simulink model "REG1_submodel"  (R2020a)
settings: Solver=VariableStepAuto  StartTime=0.0  StopTime=10.0  RelTol=1e-3
model workspace (MAT data in the model file):
  D1_podbor1 = 902.0676
  D1_podbor_psi = 334.133298018
  D1_podbor_y = 97.9069
  D_podbor_x = 10
  D_podbor_z = 10
  I1_podbor1 = 320.9285
  I1_podbor_psi = 2.71828630961
  I1_podbor_y = 0.6752
  I_podbor_x = 50
  I_podbor_z = 50
  P1_podbor1 = 7509.4
  P1_podbor_psi = 848.547345881
  P1_podbor_y = 264.9363
  P_podbor_x = 50
  P_podbor_z = 50
  theta_1_P_param = Simulink.Parameter
  theta_1_P_param.Value = 1
  theta_1_P_param.DataType = 'auto'
  theta_1_P_param.Dimensions = [1 1]
  theta_1_P_paramCopy = Simulink.Parameter
  theta_1_P_paramCopy.Value = 1
  theta_1_P_paramCopy.DataType = 'auto'
  theta_1_P_paramCopy.Dimensions = [1 1]
undefined symbols (not defined in the file or in its folder): MAV, setup_pid
libraries: simulink x26, checkpacklib x2, dspsigattribs x1
settings Model: Creator=Tamer  LastModifiedBy=Tamer
settings SolverCC: ZeroCrossControl=DisableAll
settings DataIOCC: SaveOutput=off  SaveTime=off
settings GRTTargetCC: CombineOutputUpdateFcns=off  MatFileLogging=off

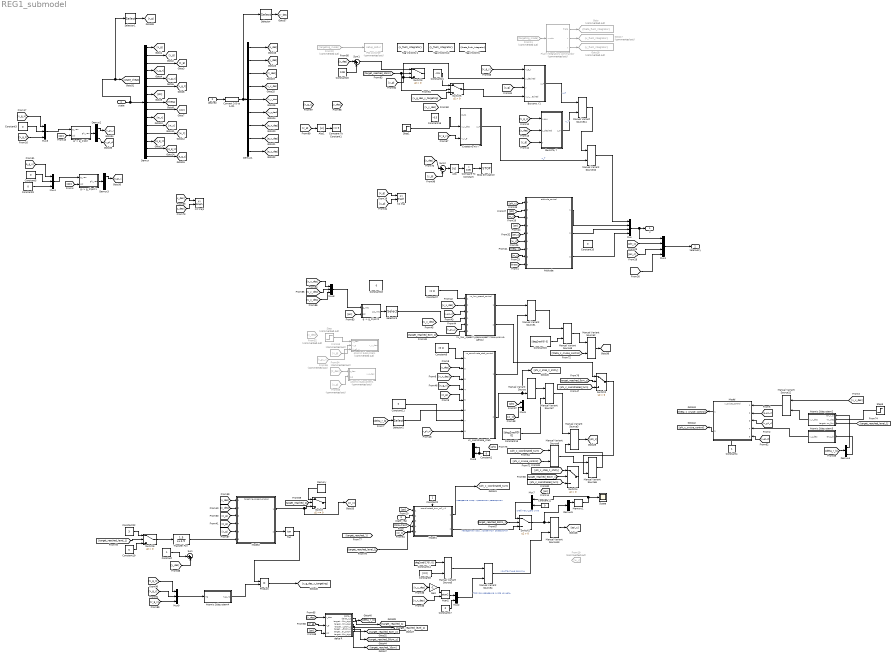
== system REG1_submodel ==
  state : Inport
  desired : Inport  Port=2  PortDimensions=[3, 3]
  state_real : Inport  Port=3
  Abs : Abs
  Abs1 : Abs
  Atan2 : Trigonometry  Operator=atan2
  Atomic Subsystem : Subsystem  Commented=on  TreatAsAtomicUnit=on
  Atomic Subsystem1 : Subsystem  Commented=on  TreatAsAtomicUnit=on
  Atomic Subsystem2 : Subsystem  TreatAsAtomicUnit=on
  Atomic Subsystem3 : Subsystem  TreatAsAtomicUnit=on
  Atomic Subsystem4 : Subsystem  TreatAsAtomicUnit=on
  Attitude : ModelReference  ModelNameDialog=attitude_control.slx  SimulationMode=Normal  ModelReferenceVersion=1.4
      settings: PortSchema="{\"entries\":[{\"content\":{\"sides\":[{\"content\":{\"connectorIds\":[\"In1\",\"In3\",\"In2\",\"In5\",\"In6\",\"In4\",\"In7\",\"In8\",\"In9\"]},\"type\":\"ConnectorPlacement.EquallySpacedRectSide\",\"uuid\":\"dbfcd847-4d65-4f0c-929f-179268b7fffa\"},{\"content\":{\"connectorIds\":[\"Out1\",\"Out2\",\"Out3\"],\"side\":\"RIGHT\"},\"type\":\"ConnectorPlacement.EquallySpacedRectSide\",\"uuid\":\"137158cb-e778-43b1-aea9-7a9702fa9882\"},{\"content\":{\"connectorIds\":[],\"side\":\"TOP\"},\"type\":\"ConnectorPlacement.EquallySpacedRectSide\",\"uuid\":\"f273673a-c2d4-42d6-9618-744ed2053ba7\"}]},\"type\":\"ConnectorPlacement.EquallySpacedConnector\",\"uuid\":\"b65e5f15-660d-4a08-8639-804897e62202\"}],\"packageUris\":[\"http://schema.mathworks.com/mf0/Connector/19700101\"],\"version\":\"1.0\"}"
  Compare To Constant : simulink/Logic and Bit Operations/Compare To Constant  relop=<  const=0.05  OutDataTypeStr=boolean
  Compare To Constant1 : simulink/Logic and Bit Operations/Compare To Constant  relop=<=  const=6  OutDataTypeStr=boolean
  Constant : Constant
  Constant{1,3,5,9..12,17..18} (9 alike) : Constant  Value=0
  Constant13 : Constant  Value=[deg2rad(0) 0]
  Constant14 : Constant  Value=[deg2rad(170); 0]
  Constant15 : Constant  Value=[deg2rad(0) 0]
  Constant16 : Constant  Value=-0.5
  Constant19 : Constant  Value=5
  Constant2 : Constant
  Constant20 : Constant  Value=0.08
  Constant21 : Constant  Value=-0.5
  Constant22 : Constant  Value=3
  Constant4 : Constant
  Constant6 : Constant  Value=[0 1]
  Constant7 : Constant  Value=[1 1]
  Constant8 : Constant  Value=[0 0]
  Convert 2-D to 1-D1 : dspsigattribs/Convert 2-D to 1-D
      settings: SourceProductBaseCode=DS
  Demux : Demux  Outputs=15
  Demux1 : Demux  Outputs=9
  Demux2 : Demux  Outputs=3
  Demux3 : Demux  Outputs=3
  Demux4 : Demux  Outputs=3
  Demux5 : Demux  Outputs=2
  Flush integrators commandor : Subsystem  Commented=on
  From11 : From  Commented=on  GotoTag=targeting_mode  TagVisibility=global
  From19 : From  Commented=on  GotoTag=w_y
  From22 : From  Commented=on  GotoTag=targeting_mode  TagVisibility=global
  From52 : From  Commented=on  GotoTag=x_des
  From53 : From  Commented=on  GotoTag=x_g
  From54 : From  Commented=on  GotoTag=z_des
  From55 : From  Commented=on  GotoTag=z_g
  From56 : From  Commented=on  GotoTag=v_g1_x
  Gain : Gain  Gain=-1
  Goto : Goto  Commented=on  GotoTag=theta_flush_integrator  TagVisibility=scoped
  Goto17 : Goto  Commented=on  GotoTag=x_flush_integrator  TagVisibility=scoped
  Goto18 : Goto  Commented=on  GotoTag=y_flush_integrator  TagVisibility=scoped
  Manual Variant Source{,1,4,7..8,10..11,13} (8 alike) : simulink/Signal Routing/Manual Variant Source  NumChoices=2  LabelModeActiveChoice=V_1
  Manual Variant Source{2..3,5..6,9,12} (6 alike) : simulink/Signal Routing/Manual Variant Source  NumChoices=2  LabelModeActiveChoice=V_2
  Memory : Memory
  Memory1 : Memory
  Model : ModelReference  ModelNameDialog=v_cruise_control.slx  SimulationMode=Normal  ModelReferenceVersion=1.37  EnablePortName=Enable  EnablePortStatesWhenEnabling=held
  Model1 : ModelReference  ModelNameDialog=coordinated_turn_roll_v1.slx  SimulationMode=Normal  ModelReferenceVersion=1.128  EnablePortName=Enable  EnablePortStatesWhenEnabling=held
  Model2 : ModelReference  ModelNameDialog=targeting_speed_angles.slx  SimulationMode=Normal  ModelReferenceVersion=1.18
  Mux : Mux
  Mux1 : Mux
  Mux{2,5..7} (4 alike) : Mux  Inputs=2
  Mux{3..4,8..9} (4 alike) : Mux  Inputs=3
  PID switcher : MATLABFcn  Commented=on  MATLABFcn=setup_pid(u)  OutputDimensions=0  Output1D=off
  Product : Product
  Scope : Scope
  Selector : Selector  InputPortWidth=9  IndexOptions=Index vector (dialog)  Indices=[1:3]  OutputSizes=1
  Selector1 : Selector  InputPortWidth=15  IndexOptions=Index vector (dialog)  Indices=[1:3]  OutputSizes=1
  Selector2 : Selector  InputPortWidth=3  IndexOptions=Index vector (dialog)  Indices=[3]  OutputSizes=1
  Selector3 : Selector  InputPortWidth=3  IndexOptions=Index vector (dialog)  Indices=[3]  OutputSizes=1
  Step : Step  Commented=on  Time=0.2  After=5  SampleTime=0
  Step1 : Step  Time=3  Before=-1  After=0  SampleTime=0
  Step3 : Step  Time=0  After=20  SampleTime=0
  Stop Simulation : Stop
  Sum : Sum  Inputs=|++
  Sum1 : Sum  Inputs=|++
  Sum2 : Sum  Inputs=|+-
  Switch : Switch  Criteria=u2 ~= 0
  Switch{1..6} (6 alike) : Switch  Criteria=u2 > Threshold
  Tag Visibility : GotoTagVisibility  GotoTag=theta_flush_integrator
  Tag Visibility1 : GotoTagVisibility  GotoTag=x_flush_integrator
  Tag Visibility2 : GotoTagVisibility  GotoTag=y_flush_integrator
  Tan : Trigonometry  Operator=tan
  Transfer Fcn : TransferFcn  Numerator=[1.5]  Denominator=[1 1.5]
  XZ traj : simulink/Sinks/XY Graph  xmin=-2  xmax=20  ymin=-2  ymax=20  st=-1
  XZ traj1 : simulink/Sinks/XY Graph  xmin=20  xmax=80  ymin=20  ymax=80  st=-1
  delta R : Subsystem  TreatAsAtomicUnit=on
  "g -> g_1(psi)" : MATLAB Function  TreatAsAtomicUnit=on
  "g -> g_1(psi)1" : MATLAB Function  TreatAsAtomicUnit=on
  "g -> g_1(psi)2" : MATLAB Function  TreatAsAtomicUnit=on
  xz_coordinate_stab : ModelReference  ModelNameDialog=xz_coordinate_stab_control.slx  SimulationMode=Normal  ModelReferenceVersion=1.10
  zx_low_speed (удерживает позицию на ветру) : ModelReference  ModelNameDialog=xz_low_speed_control.slx  SimulationMode=Normal  ModelReferenceVersion=1.12
  "Высота, Y" : Subsystem
      settings: PortSchema="{\"entries\":[{\"content\":{\"sides\":[{\"content\":{\"connectorIds\":[]},\"type\":\"ConnectorPlacement.EquallySpacedRectSide\",\"uuid\":\"a258f665-a86a-4482-bd07-3187ea478656\"},{\"content\":{\"connectorIds\":[],\"side\":\"RIGHT\"},\"type\":\"ConnectorPlacement.EquallySpacedRectSide\",\"uuid\":\"4cc1ffc1-e5d7-4190-ba75-89ce977e4acc\"},{\"content\":{\"connectorIds\":[\"Out1\"],\"side\":\"TOP\"},\"type\":\"ConnectorPlacement.EquallySpacedRectSide\",\"uuid\":\"daf9489c-9fb9-498c-b344-dda7a980194c\"},{\"content\":{\"connectorIds\":[\"In1\",\"In2\",\"In3\"],\"side\":\"BOTTOM\"},\"type\":\"ConnectorPlacement.EquallySpacedRectSide\",\"uuid\":\"f778d476-c858-4cc3-a786-5ff47391ec3b\"}]},\"type\":\"ConnectorPlacement.EquallySpacedConnector\",\"uuid\":\"5a79eedc-deb4-47bd-85cd-0d2cb0ea5802\"}],\"packageUris\":[\"http://schema.mathworks.com/mf0/Connector/19700101\"],\"version\":\"1.0\"}"
  "Высота, Y1" : Subsystem
      settings: PortSchema="{\"entries\":[{\"content\":{\"sides\":[{\"content\":{\"connectorIds\":[]},\"type\":\"ConnectorPlacement.EquallySpacedRectSide\",\"uuid\":\"a258f665-a86a-4482-bd07-3187ea478656\"},{\"content\":{\"connectorIds\":[],\"side\":\"RIGHT\"},\"type\":\"ConnectorPlacement.EquallySpacedRectSide\",\"uuid\":\"4cc1ffc1-e5d7-4190-ba75-89ce977e4acc\"},{\"content\":{\"connectorIds\":[\"Out1\"],\"side\":\"TOP\"},\"type\":\"ConnectorPlacement.EquallySpacedRectSide\",\"uuid\":\"daf9489c-9fb9-498c-b344-dda7a980194c\"},{\"content\":{\"connectorIds\":[\"In1\",\"In2\",\"In3\",\"In4\"],\"side\":\"BOTTOM\"},\"type\":\"ConnectorPlacement.EquallySpacedRectSide\",\"uuid\":\"f778d476-c858-4cc3-a786-5ff47391ec3b\"}]},\"type\":\"ConnectorPlacement.EquallySpacedConnector\",\"uuid\":\"5a79eedc-deb4-47bd-85cd-0d2cb0ea5802\"}],\"packageUris\":[\"http://schema.mathworks.com/mf0/Connector/19700101\"],\"version\":\"1.0\"}"
  Скорость по Y : Subsystem
      settings: PortSchema="{\"entries\":[{\"content\":{\"sides\":[{\"content\":{\"connectorIds\":[]},\"type\":\"ConnectorPlacement.EquallySpacedRectSide\",\"uuid\":\"a258f665-a86a-4482-bd07-3187ea478656\"},{\"content\":{\"connectorIds\":[],\"side\":\"RIGHT\"},\"type\":\"ConnectorPlacement.EquallySpacedRectSide\",\"uuid\":\"4cc1ffc1-e5d7-4190-ba75-89ce977e4acc\"},{\"content\":{\"connectorIds\":[\"Out2\"],\"side\":\"TOP\"},\"type\":\"ConnectorPlacement.EquallySpacedRectSide\",\"uuid\":\"daf9489c-9fb9-498c-b344-dda7a980194c\"},{\"content\":{\"connectorIds\":[\"Out1\",\"In1\",\"In2\"],\"side\":\"BOTTOM\"},\"type\":\"ConnectorPlacement.EquallySpacedRectSide\",\"uuid\":\"f778d476-c858-4cc3-a786-5ff47391ec3b\"}]},\"type\":\"ConnectorPlacement.EquallySpacedConnector\",\"uuid\":\"5a79eedc-deb4-47bd-85cd-0d2cb0ea5802\"}],\"packageUris\":[\"http://schema.mathworks.com/mf0/Connector/19700101\"],\"version\":\"1.0\"}"
  u : Outport
  telemetry : Outport  Port=2
  wires:
  desired/1 -> Convert 2-D to 1-D1/1
  Demux/4 -> [v_g_x]
  Demux/15 -> [a_g_z]
  Demux/13 -> [a_g_x]
  Demux/12 -> [w_z]
  From22/1 -> PID switcher/1
  Demux/3 -> [z_g]
  Demux/6 -> [v_g_z]
  Demux1/1 -> [x_des]
  Demux1/4 -> [v_x_des]
  Demux/5 -> [v_g_y]
  Demux/2 -> [y_g]
  Demux/1 -> [x_g]
  Mux/1 -> Mux1/1, u/1
  Flush integrators commandor/1(theta) -> Goto/1
  Convert 2-D to 1-D1/1 -> Selector/1, Demux1/1
  Flush integrators commandor/3(y) -> Goto18/1
  Demux1/2 -> [y_des]
  Demux/14 -> [a_g_y]
  [psi_c] -> Mux1/3
  Demux/7 -> [phi]
  Demux1/5 -> [v_y_des]
  Constant3/1 -> Mux3/2
  Mux1/1 -> telemetry/1
  Demux1/8 -> [a_y_des]
  [psi] -> "g -> g_1(psi)"/2(psi)
  [phi_c] -> Mux1/2
  Demux1/6 -> [v_z_des]
  Mux3/1 -> "g -> g_1(psi)"/1(g_vec)
  Demux1/3 -> [z_des]
  Demux2/1 -> [v_g1_x]
  [v_g_z] -> Mux3/3
  Demux/10 -> [w_x]
  [v_g_x] -> Mux3/1
  Flush integrators commandor/2(x) -> Goto17/1
  "Высота, Y"/1(u_T) -> Manual Variant Source11/2  "u_T"
  Demux/8 -> [theta]
  Demux2/3 -> [v_g1_z]
  From11/1 -> Flush integrators commandor/1(mode)
  [y_g] -> "Высота, Y"/3(y)
  "g -> g_1(psi)"/1(g1_vec) -> Demux2/1
  Demux1/7 -> [a_x_des]
  Demux/9 -> [psi]
  [theta_c] -> Mux1/4
  Demux1/9 -> [a_z_des]
  Demux/11 -> [w_y]
  Constant7/1 -> zx_low_speed (удерживает позицию на ветру)/1
  [v_g_y] -> "Высота, Y"/1(v_g_y)
  [y_des] -> "Высота, Y"/2(y_desired)
  [v_g1_z] -> zx_low_speed (удерживает позицию на ветру)/5
  [v_g1_x] -> zx_low_speed (удерживает позицию на ветру)/3
  [v_x_des] -> xz_coordinate_stab/3
  [x_des] -> xz_coordinate_stab/2
  [x_g] -> xz_coordinate_stab/5
  [v_g_x] -> xz_coordinate_stab/4
  [v_g1_z] -> xz_coordinate_stab/8
  Constant6/1 -> xz_coordinate_stab/1
  xz_coordinate_stab/2 -> [phi_c_stab_z_shitly], Manual Variant Source/2
  xz_coordinate_stab/1 -> Manual Variant Source1/2
  zx_low_speed (удерживает позицию на ветру)/1 -> Manual Variant Source1/1
  [theta] -> Attitude/9
  [phi] -> Attitude/3
  [w_x] -> Attitude/2
  [phi_c] -> Attitude/1
  Attitude/1 -> Mux/2
  Attitude/3 -> Mux/4
  Constant4/1 -> Model/Enable
  Manual Variant Source2/1 -> [theta_c]
  [v_g1_x] -> Model/3
  Demux3/1 -> [a_g1_x]
  Constant9/1 -> Mux4/3
  [a_g_x] -> Mux4/1
  [psi] -> "g -> g_1(psi)1"/2(psi)
  Mux4/1 -> "g -> g_1(psi)1"/1(g_vec)
  Constant5/1 -> Mux4/2
  "g -> g_1(psi)1"/1(g1_vec) -> Demux3/1
  [a_g1_x] -> Model/2
  Attitude/2 -> Mux/3
  [psi] -> Model1/1
  state_real/1 -> Model1/2
  Constant2/1 -> Model1/Enable
  [psi] -> Attitude/5
  [psi_c] -> Attitude/6
  [w_y] -> Attitude/4
  [theta_c] -> Attitude/7
  [w_z] -> Attitude/8
  [x_g] -> XZ traj/1
  [z_g] -> XZ traj/2
  [v_z_des] -> Gain/1
  Gain/1 -> Atan2/1
  [v_x_des] -> Atan2/2
  Atan2/1 -> Mux2/1
  Mux2/1 -> Manual Variant Source4/2  "Прямое наведение курса на цель"
  state/1 -> Selector1/1, [state_cheat], Demux/1
  [w_x] -> Mux6/2
  [phi] -> Mux6/1
  Manual Variant Source/1 -> Manual Variant Source7/1
  Manual Variant Source7/1 -> Manual Variant Source3/1
  Constant13/1 -> Manual Variant Source7/2
  [state_cheat] -> Model1/3
  [x_des] -> Model2/1
  [z_des] -> Model2/2
  [z_g] -> Model2/4
  [x_g] -> Model2/3
  [xi_c] -> Model1/4
  From53/1 -> Atomic Subsystem/2(x_g)
  From55/1 -> Atomic Subsystem1/2(z_g)
  From54/1 -> Atomic Subsystem1/1(z_des)
  From56/1 -> Atomic Subsystem/3(V_g1_x)
  Atomic Subsystem3/1(v_z_des) -> Model/4
  [v_g1_z] -> Model/5
  Step/1 -> Atomic Subsystem/1(x_des)
  [v_x_des] -> zx_low_speed (удерживает позицию на ветру)/2
  [v_x_des] -> Manual Variant Source12/1
  Selector/1 -> [r_des]
  Selector1/1 -> [r_g]
  Model2/1 -> [xi_c], Switch/3
  Memory/1 -> Switch/1
  Model1/2 -> Switch1/3  "наведение координированным разворотом"
  Constant12/1 -> Mux7/2
  [target_reached_50cm_z] -> Switch1/2
  [delta_r_b] -> Demux4/1
  Demux4/3 -> Atomic Subsystem3/1(err_z_b)
  Demux4/1 -> Atomic Subsystem2/1(err_x_b)
  Manual Variant Source9/1 -> Manual Variant Source2/1
  Manual Variant Source1/1 -> Manual Variant Source9/1
  Constant15/1 -> Manual Variant Source9/2
  [v_g_y] -> Скорость по Y/2(v_y_g)
  Скорость по Y/2(u_T) -> Manual Variant Source10/2  "u_T"
  Manual Variant Source10/1 -> Mux/1
  Step1/1 -> Скорость по Y/1(v_y_des)
  [v_g_y] -> "Высота, Y1"/1(v_g_y)
  [y_g] -> "Высота, Y1"/3(y)
  "Высота, Y1"/1(u_T) -> Manual Variant Source11/1  "u_T"
  Manual Variant Source11/1 -> Manual Variant Source10/1
  Manual Variant Source12/1 -> Model/1
  Atomic Subsystem2/1(v_x_des) -> Manual Variant Source12/2
  Constant17/1 -> Mux2/2
  Constant14/1 -> Manual Variant Source5/1
  Constant8/1 -> Manual Variant Source5/2
  Manual Variant Source13/1 -> [psi_c]
  Manual Variant Source5/1 -> Manual Variant Source4/1
  Manual Variant Source4/1 -> Manual Variant Source13/2  "константные режимы"
  delta R/2(delta_r_b) -> [delta_r_b]
  [psi] -> delta R/3(psi)
  [r_des] -> delta R/1(r_des)
  [r_g] -> delta R/2(r_g)
  delta R/3(target_near_1.5m_sign) -> [target_reached_1]
  [target_reached_1] -> Switch/2
  [phi_c_coordinated_turn] -> Manual Variant Source8/1
  Model/2 -> [phi_c_cruise_control]
  [phi_c_cruise_control] -> Manual Variant Source8/2
  Manual Variant Source3/1 -> [phi_c]
  Model/1 -> [theta_c_cruise_control]
  [theta_c_cruise_control] -> Manual Variant Source2/2
  [x_des] -> XZ traj1/1
  [z_des] -> XZ traj1/2
  Step3/1 -> Atomic Subsystem2/2(Vx_des)
  delta R/4(target_near_3m_sign) -> [target_reached_level_1]
  [target_reached_level_1] -> Atomic Subsystem2/3(target_near_3m)
  Model1/1 -> [phi_c_coordinated_turn]  "наведение координированным разворотом"
  Constant1/1 -> Mux5/1, Mux5/2
  [target_reached_5cm_z] -> Switch2/2
  delta R/5(target_near_5cm_z) -> [target_reached_5cm_z]
  Mux7/1 -> Switch1/1  "стаб текущего угла"
  [target_reached_level_1] -> Model1/5
  Switch1/1 -> Demux5/1, Manual Variant Source13/1
  delta R/6(target_near_50cm_z) -> [target_reached_50cm_z]
  Manual Variant Source6/1 -> Manual Variant Source3/2
  Manual Variant Source8/1 -> Manual Variant Source6/1
  [target_reached_50cm_z] -> Switch4/2
  [phi_c_stab_z_shitly] -> Switch4/1
  [phi_c_coordinated_turn] -> Switch4/3
  Demux5/1 -> Memory1/1
  Memory1/1 -> Scope/1, Mux7/1
  Constant11/1 -> xz_coordinate_stab/7
  [delta_r_b] -> Selector2/1
  Selector2/1 -> xz_coordinate_stab/6
  zx_low_speed (удерживает позицию на ветру)/2 -> Switch2/1
  [phi_c_coordinated_turn] -> Switch2/3
  [target_reached_5cm_z] -> zx_low_speed (удерживает позицию на ветру)/6
  Switch2/1 -> Manual Variant Source6/2
  [psi] -> "g -> g_1(psi)2"/2(psi)
  [v_x_des] -> Mux8/1
  [v_y_des] -> Mux8/2
  [v_z_des] -> Mux8/3
  Mux8/1 -> "g -> g_1(psi)2"/1(g_vec)
  "g -> g_1(psi)2"/1(g1_vec) -> Selector3/1
  Selector3/1 -> zx_low_speed (удерживает позицию на ветру)/4
  [y_g] -> Model2/5
  [v_g_y] -> Mux9/2
  Mux9/1 -> Atomic Subsystem4/1(Vg)
  [v_g_z] -> Mux9/3
  [v_g_x] -> Mux9/1
  Model2/2 -> Tan/1
  Atomic Subsystem4/1(V_g_xz) -> Product/2
  Tan/1 -> Product/1
  Switch5/1 -> "Высота, Y1"/4(v_y_desired)
  [y_g] -> "Высота, Y1"/2(y_desired), Switch3/3
  [target_reached_10cm] -> Switch5/2, Switch3/2
  Sum1/1 -> Switch3/1
  [v_g_des_y_targeting] -> Switch5/3
  delta R/7(target_near_10cm) -> [target_reached_10cm]
  [y_des] -> Sum1/1
  Constant20/1 -> Sum1/2
  [y_des] -> Sum/2
  Constant/1 -> Sum/1
  Sum2/1 -> Abs/1
  [y_des] -> Sum2/1
  [y_g] -> Sum2/2
  Abs/1 -> Compare To Constant/1
  Constant21/1 -> Switch5/1
  Abs1/1 -> Compare To Constant1/1
  [y_g] -> Abs1/1
  Constant22/1 -> Switch6/1
  Constant19/1 -> Switch6/3
  [target_reached_level_1] -> Switch6/2
  Compare To Constant/1 -> Stop Simulation/1
  Switch6/1 -> Transfer Fcn/1
  Transfer Fcn/1 -> Model2/6
  Product/1 -> [v_g_des_y_targeting]

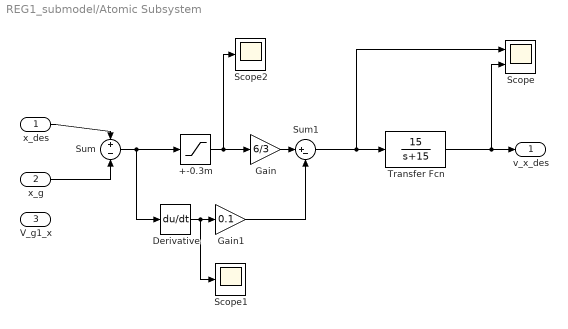
== system REG1_submodel/Atomic Subsystem ==
  x_des : Inport
  x_g : Inport  Port=2
  V_g1_x : Inport  Port=3
  +-0.3m : Saturate  UpperLimit=3  LowerLimit=-3
  Derivative : Derivative
  Gain : Gain  Gain=6/3
  Gain1 : Gain  Gain=0.1
  Scope : Scope  NumInputPorts=2
  Scope1 : Scope
  Scope2 : Scope
  Sum : Sum  Inputs=+-
  Sum1 : Sum  Inputs=|+-
  Transfer Fcn : TransferFcn  Numerator=[15]  Denominator=[1 15]
  v_x_des : Outport
  wires:
  x_des/1 -> Sum/1
  x_g/1 -> Sum/2
  +-0.3m/1 -> Scope2/1, Gain/1
  Gain/1 -> Sum1/1
  Sum1/1 -> Transfer Fcn/1, Scope/1
  Gain1/1 -> Sum1/2
  Sum/1 -> Derivative/1, +-0.3m/1
  Derivative/1 -> Scope1/1, Gain1/1
  Transfer Fcn/1 -> Scope/2, v_x_des/1

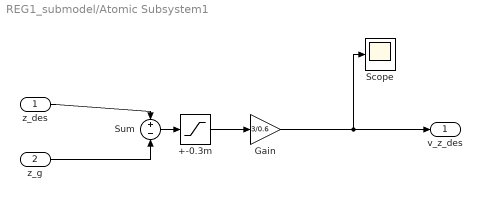
== system REG1_submodel/Atomic Subsystem1 ==
  z_des : Inport
  z_g : Inport  Port=2
  +-0.3m : Saturate  UpperLimit=0.6  LowerLimit=-0.6
  Gain : Gain  Gain=3/0.6
  Scope : Scope
  Sum : Sum  Inputs=+-
  v_z_des : Outport
  wires:
  z_des/1 -> Sum/1
  z_g/1 -> Sum/2
  Sum/1 -> +-0.3m/1
  +-0.3m/1 -> Gain/1
  Gain/1 -> Scope/1, v_z_des/1

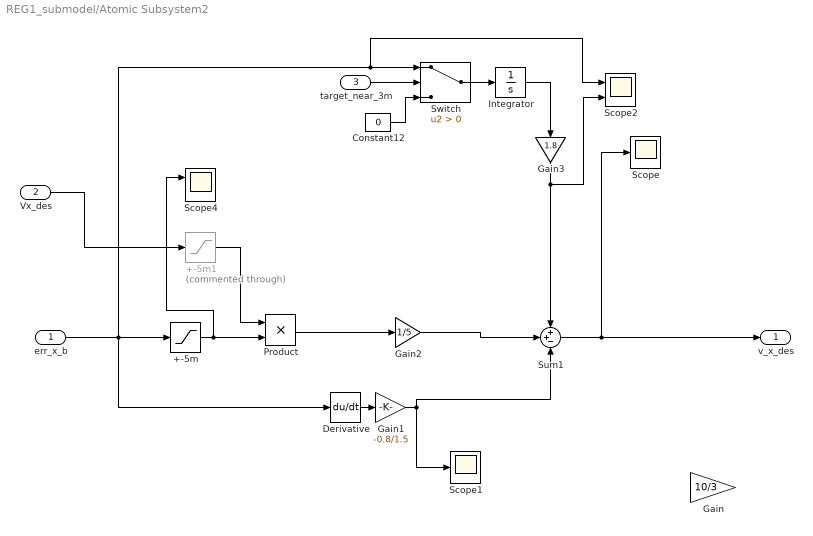
== system REG1_submodel/Atomic Subsystem2 ==
  err_x_b : Inport
  Vx_des : Inport  Port=2
  target_near_3m : Inport  Port=3
  +-5m : Saturate  UpperLimit=5  LowerLimit=-5
  +-5m1 : Saturate  Commented=through  UpperLimit=20  LowerLimit=-20
  Constant12 : Constant  Value=0
  Derivative : Derivative
  Gain : Gain  Gain=10/3
  Gain1 : Gain  Gain=-0.8/1.5
  Gain2 : Gain  Gain=1/5
  Gain3 : Gain  Gain=1.8
  Integrator : Integrator
  Product : Product
  Scope : Scope
  Scope1 : Scope
  Scope2 : Scope  NumInputPorts=2
  Scope4 : Scope  NumInputPorts=2
  Sum1 : Sum  Inputs=++-
  Switch : Switch  Criteria=u2 > Threshold
  v_x_des : Outport
  wires:
  +-5m/1 -> Scope4/1, Product/2
  err_x_b/1 -> Scope2/1, Switch/1, +-5m/1, Derivative/1
  Gain1/1 -> Sum1/3, Scope1/1
  Derivative/1 -> Gain1/1
  Product/1 -> Gain2/1
  Sum1/1 -> v_x_des/1, Scope/1
  target_near_3m/1 -> Switch/2
  Switch/1 -> Integrator/1
  Constant12/1 -> Switch/3
  Gain3/1 -> Sum1/1, Scope2/2
  Integrator/1 -> Gain3/1
  Gain2/1 -> Sum1/2
  Vx_des/1 -> +-5m1/1
  +-5m1/1 -> Product/1

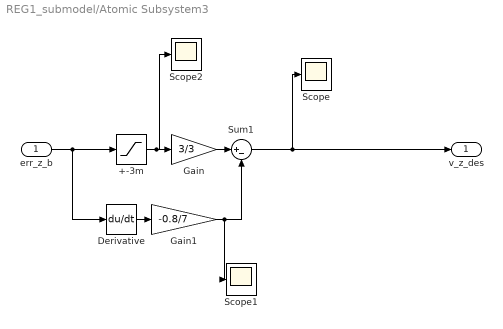
== system REG1_submodel/Atomic Subsystem3 ==
  err_z_b : Inport
  +-3m : Saturate  UpperLimit=3  LowerLimit=-3
  Derivative : Derivative
  Gain : Gain  Gain=3/3
  Gain1 : Gain  Gain=-0.8/7
  Scope : Scope
  Scope1 : Scope
  Scope2 : Scope
  Sum1 : Sum  Inputs=|+-
  v_z_des : Outport
  wires:
  +-3m/1 -> Scope2/1, Gain/1
  Gain/1 -> Sum1/1
  Sum1/1 -> v_z_des/1, Scope/1
  err_z_b/1 -> Derivative/1, +-3m/1
  Gain1/1 -> Sum1/2, Scope1/1
  Derivative/1 -> Gain1/1

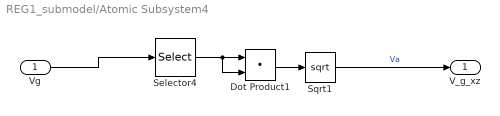
== system REG1_submodel/Atomic Subsystem4 ==
  Vg : Inport
  Dot Product1 : DotProduct  InputSameDT=on  OutDataTypeStr=Inherit: Inherit via internal rule
  Selector4 : Selector  InputPortWidth=3  IndexOptions=Index vector (dialog)  Indices=[1 3]  OutputSizes=1
  Sqrt1 : Sqrt  SaturateOnIntegerOverflow=on
  V_g_xz : Outport
  wires:
  Selector4/1 -> Dot Product1/2, Dot Product1/1
  Dot Product1/1 -> Sqrt1/1
  Vg/1 -> Selector4/1
  Sqrt1/1 -> V_g_xz/1  "Va"

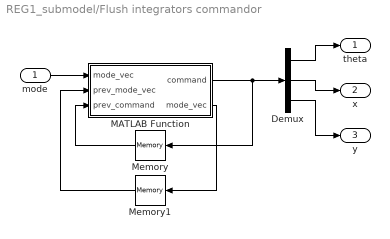
== system REG1_submodel/Flush integrators commandor ==
  mode : Inport
  Demux : Demux  Outputs=3
  MATLAB Function : MATLAB Function  TreatAsAtomicUnit=on
  Memory : Memory  InitialCondition=[0 0 0]'
  Memory1 : Memory  InitialCondition=[0 0]'
  theta : Outport
  x : Outport  Port=2
  y : Outport  Port=3
  wires:
  mode/1 -> MATLAB Function/1("mode_vec ")
  MATLAB Function/1(command) -> Memory/1, Demux/1
  Memory/1 -> MATLAB Function/3(prev_command)
  Demux/1 -> theta/1
  Demux/2 -> x/1
  Demux/3 -> y/1
  MATLAB Function/2(mode_vec) -> Memory1/1
  Memory1/1 -> MATLAB Function/2(prev_mode_vec)

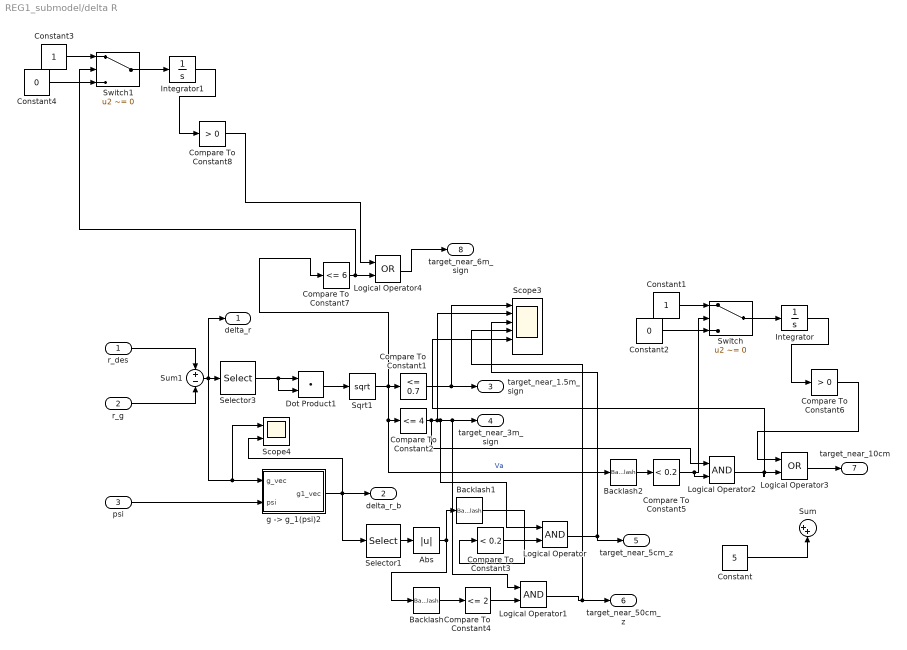
== system REG1_submodel/delta R ==
  r_des : Inport
  r_g : Inport  Port=2
  psi : Inport  Port=3
  Abs : Abs
  Backlash : Backlash  InitialOutput=2
  Backlash1 : Backlash  BacklashWidth=0.1  InitialOutput=0.2
  Backlash2 : Backlash  BacklashWidth=0.1  InitialOutput=0.25
  Compare To Constant1 : simulink/Logic and Bit Operations/Compare To Constant  relop=<=  const=0.7  OutDataTypeStr=boolean
  Compare To Constant2 : simulink/Logic and Bit Operations/Compare To Constant  relop=<=  const=4  OutDataTypeStr=boolean
  Compare To Constant3 : simulink/Logic and Bit Operations/Compare To Constant  relop=<  const=0.2  OutDataTypeStr=boolean
  Compare To Constant4 : simulink/Logic and Bit Operations/Compare To Constant  relop=<=  const=2  OutDataTypeStr=boolean
  Compare To Constant5 : simulink/Logic and Bit Operations/Compare To Constant  relop=<  const=0.2  OutDataTypeStr=boolean
  Compare To Constant6 : simulink/Logic and Bit Operations/Compare To Constant  relop=>  const=0  OutDataTypeStr=boolean
  Compare To Constant7 : simulink/Logic and Bit Operations/Compare To Constant  relop=<=  const=6  OutDataTypeStr=boolean
  Compare To Constant8 : simulink/Logic and Bit Operations/Compare To Constant  relop=>  const=0  OutDataTypeStr=boolean
  Constant : Constant  Value=5
  Constant1 : Constant
  Constant2 : Constant  Value=0
  Constant3 : Constant
  Constant4 : Constant  Value=0
  Dot Product1 : DotProduct  InputSameDT=on  OutDataTypeStr=Inherit: Inherit via internal rule
  Integrator : Integrator
  Integrator1 : Integrator
  Logical Operator : Logic  AllPortsSameDT=off  OutDataTypeStr=boolean
  Logical Operator1 : Logic  AllPortsSameDT=off  OutDataTypeStr=boolean
  Logical Operator2 : Logic  AllPortsSameDT=off  OutDataTypeStr=boolean
  Logical Operator3 : Logic  Operator=OR  AllPortsSameDT=off  OutDataTypeStr=boolean
  Logical Operator4 : Logic  Operator=OR  AllPortsSameDT=off  OutDataTypeStr=boolean
  Scope3 : Scope  NumInputPorts=6
  Scope4 : Scope  NumInputPorts=2
  Selector1 : Selector  InputPortWidth=3  IndexOptions=Index vector (dialog)  Indices=[3]  OutputSizes=1
  Selector3 : Selector  InputPortWidth=3  IndexOptions=Index vector (dialog)  Indices=[1 3]  OutputSizes=1
  Sqrt1 : Sqrt  SaturateOnIntegerOverflow=on
  Sum : Sum  Inputs=|++
  Sum1 : Sum  Inputs=+-
  Switch : Switch  Criteria=u2 ~= 0
  Switch1 : Switch  Criteria=u2 ~= 0
  "g -> g_1(psi)2" : MATLAB Function  TreatAsAtomicUnit=on
  delta_r : Outport
  delta_r_b : Outport  Port=2
  target_near_1.5m_sign : Outport  Port=3
  target_near_3m_sign : Outport  Port=4
  target_near_5cm_z : Outport  Port=5
  target_near_50cm_z : Outport  Port=6
  target_near_10cm : Outport  Port=7
  target_near_6m_sign : Outport  Port=8
  wires:
  r_g/1 -> Sum1/2
  Selector3/1 -> Dot Product1/2, Dot Product1/1
  Dot Product1/1 -> Sqrt1/1
  psi/1 -> "g -> g_1(psi)2"/2(psi)
  Sum1/1 -> delta_r/1, Selector3/1, Scope4/1, "g -> g_1(psi)2"/1(g_vec)
  Sqrt1/1 -> Compare To Constant7/1, Backlash2/1, Compare To Constant2/1, Compare To Constant1/1  "Va"
  "g -> g_1(psi)2"/1(g1_vec) -> Selector1/1, delta_r_b/1, Scope4/2
  r_des/1 -> Sum1/1
  Compare To Constant1/1 -> Scope3/1, target_near_1.5m_sign/1
  Compare To Constant2/1 -> Logical Operator2/1, target_near_3m_sign/1, Logical Operator1/1, Logical Operator/1, Scope3/2
  Selector1/1 -> Abs/1
  Logical Operator/1 -> target_near_5cm_z/1, Scope3/3
  Compare To Constant3/1 -> Logical Operator/2
  Compare To Constant4/1 -> Logical Operator1/2
  Logical Operator1/1 -> Scope3/4, target_near_50cm_z/1
  Abs/1 -> Backlash1/1, Backlash/1
  Backlash/1 -> Compare To Constant4/1
  Backlash1/1 -> Compare To Constant3/1
  Compare To Constant5/1 -> Switch/2, Logical Operator2/2
  Logical Operator2/1 -> Logical Operator3/2, Scope3/5
  Backlash2/1 -> Compare To Constant5/1
  Constant/1 -> Sum/2
  Switch/1 -> Integrator/1
  Constant1/1 -> Switch/1
  Constant2/1 -> Switch/3
  Logical Operator3/1 -> target_near_10cm/1
  Integrator/1 -> Compare To Constant6/1
  Compare To Constant6/1 -> Logical Operator3/1
  Compare To Constant7/1 -> Logical Operator4/2, Switch1/2
  Constant3/1 -> Switch1/1
  Constant4/1 -> Switch1/3
  Integrator1/1 -> Compare To Constant8/1
  Switch1/1 -> Integrator1/1
  Compare To Constant8/1 -> Logical Operator4/1
  Logical Operator4/1 -> target_near_6m_sign/1

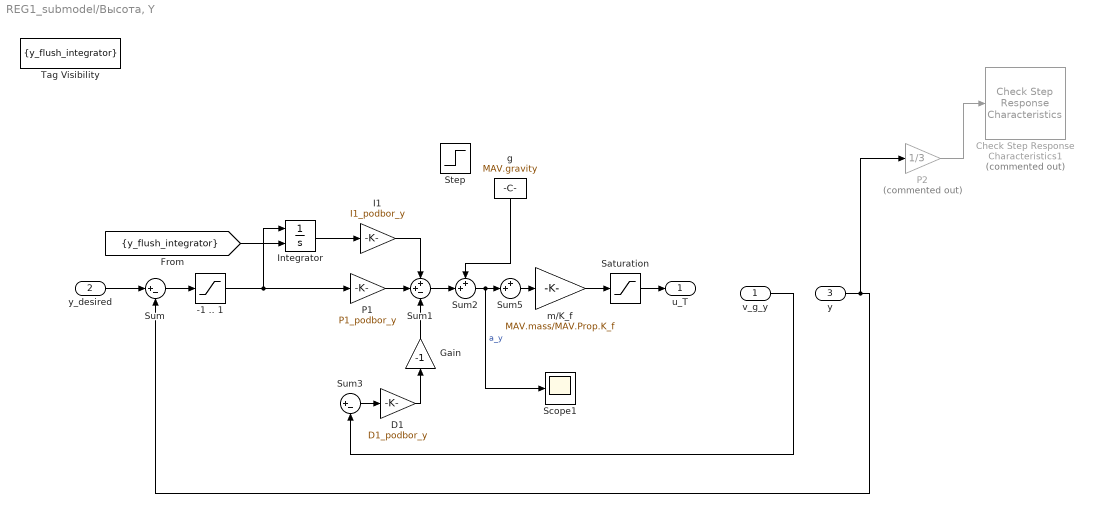
== system REG1_submodel/Высота, Y ==
  v_g_y : Inport
  y_desired : Inport  Port=2
  y : Inport  Port=3
  -1 .. 1 : Saturate  UpperLimit=1  LowerLimit=-1
  Check Step Response Characteristics1 : checkpacklib/Check Step Response  Characteristics  Commented=on  InstantiateOnLoad=on  enabled=off  stopWhenAssertionFail=off  export=off  ViewDlgPos=[299 89 1306 720]  OpenViewOnLoad=off  LaunchViewOnOpen=off  TimeUnits=seconds  EnableStepResponseBound=on  InitialValue=0  FinalValue=1  StepTime=1  RiseTime=0.7  PercentRise=80  SettlingTime=1  PercentSettling=1  PercentOvershoot=10  PercentUndershoot=1
      settings: SourceProductBaseCode=CT,ID,MT,SO
  D1 : Gain  Gain=D1_podbor_y
  Gain : Gain  Gain=-1
  I1 : Gain  Gain=I1_podbor_y
  Integrator : Integrator  ExternalReset=either
  P1 : Gain  Gain=P1_podbor_y
  P2 : Gain  Commented=on  Gain=1/3
  Saturation : Saturate  UpperLimit=4*(MAV.Motor.Nmax*0.5)^2  LowerLimit=0
  Scope1 : Scope
  Step : Step  Time=3  Before=9.81  SampleTime=0
  Sum : Sum  Inputs=|+-
  Sum1 : Sum  Inputs=++-
  Sum2 : Sum  Inputs=++|
  Sum3 : Sum  Inputs=|+-
  Sum5 : Sum  Inputs=++|
  Tag Visibility : GotoTagVisibility  GotoTag=y_flush_integrator
  g : Constant  Value=MAV.gravity
  m/K_f : Gain  Gain=MAV.mass/MAV.Prop.K_f
  u_T : Outport
  wires:
  Integrator/1 -> I1/1
  I1/1 -> Sum1/1
  P1/1 -> Sum1/2
  v_g_y/1 -> Sum3/2
  Sum1/1 -> Sum2/2
  Saturation/1 -> u_T/1
  Sum3/1 -> D1/1
  D1/1 -> Gain/1
  [y_flush_integrator] -> Integrator/2
  Gain/1 -> Sum1/3
  Sum/1 -> -1 .. 1/1
  -1 .. 1/1 -> P1/1, Integrator/1
  y_desired/1 -> Sum/1
  y/1 -> P2/1, Sum/2
  P2/1 -> Check Step Response Characteristics1/1
  Sum2/1 -> Scope1/1, Sum5/2  "a_y"
  Sum5/1 -> m/K_f/1
  g/1 -> Sum2/1
  m/K_f/1 -> Saturation/1

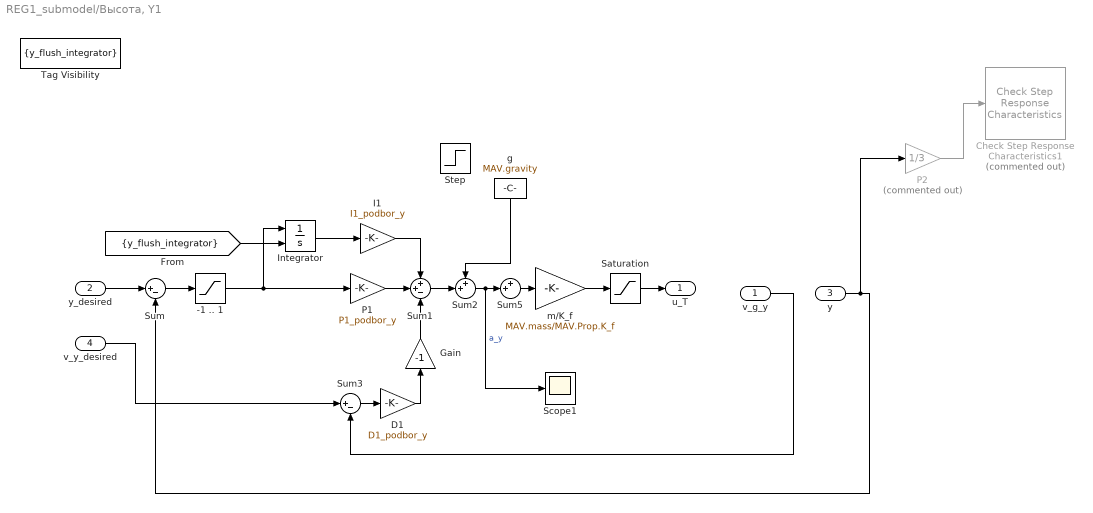
== system REG1_submodel/Высота, Y1 ==
  v_g_y : Inport
  y_desired : Inport  Port=2
  y : Inport  Port=3
  v_y_desired : Inport  Port=4
  -1 .. 1 : Saturate  UpperLimit=1  LowerLimit=-1
  Check Step Response Characteristics1 : checkpacklib/Check Step Response  Characteristics  Commented=on  InstantiateOnLoad=on  enabled=off  stopWhenAssertionFail=off  export=off  ViewDlgPos=[299 89 1306 720]  OpenViewOnLoad=off  LaunchViewOnOpen=off  TimeUnits=seconds  EnableStepResponseBound=on  InitialValue=0  FinalValue=1  StepTime=1  RiseTime=0.7  PercentRise=80  SettlingTime=1  PercentSettling=1  PercentOvershoot=10  PercentUndershoot=1
      settings: SourceProductBaseCode=CT,ID,MT,SO
  D1 : Gain  Gain=D1_podbor_y
  Gain : Gain  Gain=-1
  I1 : Gain  Gain=I1_podbor_y
  Integrator : Integrator  ExternalReset=either
  P1 : Gain  Gain=P1_podbor_y
  P2 : Gain  Commented=on  Gain=1/3
  Saturation : Saturate  UpperLimit=4*(MAV.Motor.Nmax*0.5)^2  LowerLimit=0
  Scope1 : Scope
  Step : Step  Time=3  Before=9.81  SampleTime=0
  Sum : Sum  Inputs=|+-
  Sum1 : Sum  Inputs=++-
  Sum2 : Sum  Inputs=++|
  Sum3 : Sum  Inputs=|+-
  Sum5 : Sum  Inputs=++|
  Tag Visibility : GotoTagVisibility  GotoTag=y_flush_integrator
  g : Constant  Value=MAV.gravity
  m/K_f : Gain  Gain=MAV.mass/MAV.Prop.K_f
  u_T : Outport
  wires:
  Integrator/1 -> I1/1
  I1/1 -> Sum1/1
  P1/1 -> Sum1/2
  v_g_y/1 -> Sum3/2
  Sum1/1 -> Sum2/2
  Saturation/1 -> u_T/1
  Sum3/1 -> D1/1
  D1/1 -> Gain/1
  [y_flush_integrator] -> Integrator/2
  Gain/1 -> Sum1/3
  Sum/1 -> -1 .. 1/1
  -1 .. 1/1 -> P1/1, Integrator/1
  y_desired/1 -> Sum/1
  y/1 -> P2/1, Sum/2
  P2/1 -> Check Step Response Characteristics1/1
  Sum2/1 -> Scope1/1, Sum5/2  "a_y"
  Sum5/1 -> m/K_f/1
  g/1 -> Sum2/1
  m/K_f/1 -> Saturation/1
  v_y_desired/1 -> Sum3/1

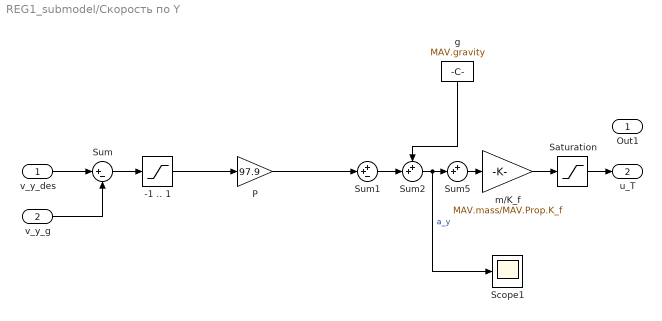
== system REG1_submodel/Скорость по Y ==
  v_y_des : Inport
  v_y_g : Inport  Port=2
  -1 .. 1 : Saturate  UpperLimit=1  LowerLimit=-1
  P : Gain  Gain=97.9
  Saturation : Saturate  UpperLimit=4*(MAV.Motor.Nmax*0.5)^2  LowerLimit=0
  Scope1 : Scope
  Sum : Sum  Inputs=|+-
  Sum1 : Sum  Inputs=++-
  Sum2 : Sum  Inputs=++|
  Sum5 : Sum  Inputs=++|
  g : Constant  Value=MAV.gravity
  m/K_f : Gain  Gain=MAV.mass/MAV.Prop.K_f
  Out1 : Outport
  u_T : Outport  Port=2
  wires:
  P/1 -> Sum1/2
  Sum1/1 -> Sum2/2
  Saturation/1 -> u_T/1
  Sum/1 -> -1 .. 1/1
  -1 .. 1/1 -> P/1
  v_y_des/1 -> Sum/1
  Sum2/1 -> Scope1/1, Sum5/2  "a_y"
  Sum5/1 -> m/K_f/1
  g/1 -> Sum2/1
  v_y_g/1 -> Sum/2
  m/K_f/1 -> Saturation/1

== matlab function REG1_submodel/g -> g_1(psi) ==
  data: g_vec input; g1_vec output; psi input
% Поворот вектора глобальной СК в полусвязанную на угол рыскания
function g1_vec = fcn(g_vec, psi)

c_p = cos(psi); s_p = sin(psi);
R = [c_p 0 -s_p; 0 1 0; s_p 0 c_p];
g1_vec = R * g_vec;

== matlab function REG1_submodel/g -> g_1(psi)1 ==
  data: g_vec input; g1_vec output; psi input
% Поворот вектора глобальной СК в полусвязанную на угол рыскания
function g1_vec = fcn(g_vec, psi)

c_p = cos(psi); s_p = sin(psi);
R = [c_p 0 -s_p; 0 1 0; s_p 0 c_p];
g1_vec = R * g_vec;

== matlab function REG1_submodel/g -> g_1(psi)2 ==
  data: g_vec input; g1_vec output; psi input
% Поворот вектора глобальной СК в полусвязанную на угол рыскания
function g1_vec = fcn(g_vec, psi)

c_p = cos(psi); s_p = sin(psi);
R = [c_p 0 -s_p; 0 1 0; s_p 0 c_p];
g1_vec = R * g_vec;

== matlab function REG1_submodel/delta R/g -> g_1(psi)2 ==
  data: g_vec input; g1_vec output; psi input
% Поворот вектора глобальной СК в полусвязанную на угол рыскания
function g1_vec = fcn(g_vec, psi)

c_p = cos(psi); s_p = sin(psi);
R = [c_p 0 -s_p; 0 1 0; s_p 0 c_p];
g1_vec = R * g_vec;

== matlab function REG1_submodel/Flush integrators commandor/MATLAB Function ==
  data: mode_vec input; prev_mode_vec input; command output; prev_command input; mode_vec output
function [command, mode_vec]  = fcn(mode_vec, prev_mode_vec, prev_command)
    command = prev_command;
%     persistent prev_mode;
%     if isempty(prev_mode)
%        prev_mode = -1; 
%     end
    if prev_mode_vec == mode_vec
        return
    end
%     prev_mode = mode;
    % command: [ theta x y]
    
    mode = FlightMode(mode_vec);
    prev_mode = FlightMode(prev_mode_vec);
    phi = 1; x = 2; y = 3;
    
    % если изменился канал х
    if mode.get('x') ~= prev_mode.get('x')
        command(x) = double(~prev_command(x));
        if mode.get('x') == 0 || mode.get('x') == 1
            command(phi) = double(~prev_command(phi));
        end
    end
    
    if mode.get('y') ~= prev_mode.get('y')
        command(y) = double(~prev_command(y));
    end
    
    

%     if mode == 2 || mode == 0
%         command = double(~prev_command);
%     end
%     if mode == 3 || mode == 5
%         command(2) = double(~prev_command(2));
%     end
%     if mode == 4 || mode == 5 || mode == 6
%         command(3) = double(~prev_command(3));
%     end
